simulink model "btp_VERSION2_final"  (R2020a)
settings: Solver=VariableStepAuto  StartTime=0.0  StopTime=14000  RelTol=1e-3
PreLoadFcn:
  | building_length = 15; % m
  | building_width = 10; % m
  | building_height = 2.5; % m
  | 
  | wall_thickness = 0.2; % m
  | wall_density = 2000; % kg/m^3
  | wall_specific_heat = 840; % J/(kg*K)
  | wall_conductivity = 0.04; % W/(m*K)
  | wall_heat_transfer_coeff_internal = 25; % W/(m^2*K)
  | wall_heat_transfer_coeff_external = 35; % W/(m^2*K)
  | 
  | roof_thickness = 0.2; % m
  | roof_density = 2000; % kg/m^3
  | roof_specific_heat = 840; % J/(kg*K)
  | roof_conductivity = 0.035; % W/(m*K)
  | roof_heat_transfer_coeff_internal = 10; % W/(m^2*K)
  | roof_heat_transfer_coeff_external = 30; % W/(m^2*K)
  | 
  | floor_thickness = 0.1; % m
  | floor_conductivity = 0.15; % W/(m*K)
  | floor_heat_transfer_coeff_internal = 15; % W/(m^2*K)
  | 
  | door_area = 2*0.6; % m^2
  | 
  | duct_area = 0.1^2; % m^2
  | 
  | fan_setting_table = 0 : 4; % 1
  | fan_flow_rate_table = [0 0.08 0.12 0.16 0.2]; % kg/s
  | 
  | initial_temperature = 35; % degC
  | ground_temperature = 25; % degC
  | 
  | flow_reversal_Mach = 1e-5; % 1
InitFcn:
  | zone_volume = building_length * building_width * building_height / 4; % m^3
  | zone_flow_area = 0.7 * building_height * (building_length + building_width) / 4; % m^2
model workspace (MAT data in the model file):
  building_height = 3
  building_length = 4.4
  building_width = 4
  door_area = Simulink.Parameter
  door_area.Value = 2
  door_area.DataType = 'double'
  door_area.Dimensions = [1 1]
  duct_area = 0.02
  fan_flow_rate_table = [0 0.08 0.12 0.16 0.2]
  fan_setting_table = [0 1 2 3 4]
  floor_conductivity = 0.15
  floor_heat_transfer_coeff_internal = 15
  floor_thickness = 0.1
  flow_reversal_Mach = 1e-05
  ground_temperature = 27
  initial_temperature = 35
  roof_conductivity = 0.04
  roof_density = 2000
  roof_heat_transfer_coeff_external = 30
  roof_heat_transfer_coeff_internal = 10
  roof_specific_heat = 840
  roof_thickness = 0.2
  simlog_ssc_building_ventilation : simscape.logging.Node (value not decoded)
  tout = [0 3.15544362088e-30 8.45959628835e-09 2.5378788865e-08 3.73619145974e-08 4.93450403297e-08 6.73197289282e-08 8.52944175267e-08 1.12256450424e-07 1.39218483322e-07 1.6618051622e-07 1.93142549118e-07 ... (463 elements, 463x1)]
  wall_conductivity = 0.04
  wall_density = 2000
  wall_heat_transfer_coeff_external = 35
  wall_heat_transfer_coeff_internal = 25
  wall_specific_heat = 840
  wall_thickness = 0.2
  zone_flow_area = 9
  zone_volume = 50
undefined symbols (not defined in the file): dbresponses22S1, sigbuilder_block
libraries: fl_lib x53, nesl_utility x27, HVAC_lib x2, simulink x2, fuzblock x1
(part 1 of 2)
CloseFcn:
  | try,close(h1_ssc_building_ventilation),end
  | clear h1_ssc_building_ventilation
  | try,close(h2_ssc_building_ventilation),end
  | clear h2_ssc_building_ventilation
  | try,close(h3_ssc_building_ventilation),end
  | clear h3_ssc_building_ventilation
  | try,close(h4_ssc_building_ventilation),end
  | clear h4_ssc_building_ventilation
  | 
  | clear simlog_ssc_building_ventilation tout
  | 
  | clear building_length building_width building_height zone_volume zone_flow_area
  | clear wall_thickness wall_density wall_specific_heat wall_conductivity wall_heat_transfer_coeff_internal wall_heat_transfer_coeff_external
  | clear roof_thickness roof_density roof_specific_heat roof_conductivity roof_heat_transfer_coeff_internal roof_heat_transfer_coeff_external
  | clear floor_thickness floor_conductivity floor_heat_transfer_coeff_internal
  | clear door_area duct_area fan_setting_table fan_flow_rate_table initial_temperature ground_temperature flow_reversal_Mach
Description:
  | Building Ventilation
settings Model: OrderedModelArguments=off  Creator=MathWorks  LastModifiedBy=PRANAV REDDY
settings DataIOCC: ReturnWorkspaceOutputs=off
settings DebuggingCC: PregeneratedLibrarySubsystemCodeDiagnostic=none  ArithmeticOperatorsInVariantConditions=warning
settings SFSimCC: SimUseLocalCustomCode=off  CustomCodeUndefinedFunction=UseInterfaceOnly
settings RTWCC: RTWUseLocalCustomCode=off
settings CodeAppCC: StateflowObjectComments=on
settings SimscapeCC: SimscapeLogType=all  SimscapeLogSimulationStatistics=on  SimscapeLogName=simlog_ssc_building_ventilation  SimscapeLogDataHistory=10000

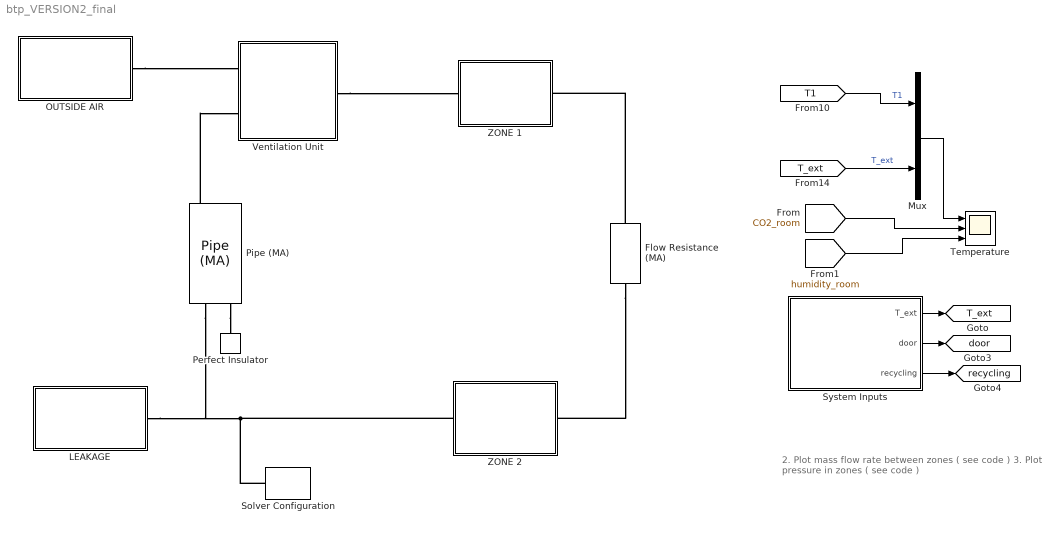
== system btp_VERSION2_final ==
  note: 2. Plot mass flow rate between zones ( see code )
      | 3. Plot pressure in zones ( see code )
  Flow Resistance (MA) : fl_lib/Moist Air/Elements/Flow Resistance (MA)  delta_p_nominal=10 Pa  mdot_nominal=0.45 kg/s  rho_nominal=1.2 kg/m^3  area=zone_flow_area m^2  laminar_fraction=1e-3
      settings: SourceProductBaseCode=SS
  LEAKAGE : Subsystem
  Mux : Mux  Inputs=2
  OUTSIDE AIR : Subsystem
  Perfect Insulator : fl_lib/Thermal/Thermal Elements/Perfect Insulator  T_specify=off  T_priority=None  T=0 K  T_nominal_specify=off  T_nominal_unit=K  T_nominal_value=1
  Pipe (MA) : fl_lib/Moist Air/Elements/Pipe (MA)  length=building_length + building_width m  area=duct_area m^2  Dh=sqrt(duct_area) m  length_add=0 m  roughness=15e-6 m  Re_lam=2000  Re_tur=4000  shape_factor=56.92  Nu_lam=2.98  RH_ws=1  time_constant=1e-3 s  moisture_trace_gas_source=foundation.enum.moisture_trace_gas_source.none  moisture_source_spec=foundation.enum.moisture_source_spec.vapor  moisture_mass_flow=0 kg/s  moisture_temperature_spec=foundation.enum.temperature_spec.atmospheric  moisture_temperature=293.15 K  trace_gas_mass_flow=0 kg/s  trace_gas_temperature_spec=foundation.enum.temperature_spec.atmospheric  trace_gas_temperature=293.15 K  p_I_specify=on  p_I_priority=High  p_I=0.101325 MPa  p_I_nominal_specify=off  p_I_nominal_unit=MPa  p_I_nominal_value=1  T_I_specify=off  T_I_priority=None  T_I=initial_temperature K  T_I_nominal_specify=off  T_I_nominal_unit=K  T_I_nominal_value=1  RH_I_specify=on  RH_I_priority=None  RH_I=0.57  RH_I_nominal_specify=off  RH_I_nominal_unit=1  RH_I_nominal_value=1  x_w_I_specify=off  x_w_I_priority=None  x_w_I=0  x_w_I_nominal_specify=off  x_w_I_nominal_unit=1  x_w_I_nominal_value=1  y_w_I_specify=off  y_w_I_priority=None  y_w_I=0  y_w_I_nominal_specify=off  y_w_I_nominal_unit=1  y_w_I_nominal_value=1  HR_I_specify=off  HR_I_priority=None  HR_I=0  HR_I_nominal_specify=off  HR_I_nominal_unit=1  HR_I_nominal_value=1  x_g_I_specify=off  x_g_I_priority=High  x_g_I=0  x_g_I_nominal_specify=off  x_g_I_nominal_unit=1  x_g_I_nominal_value=1  y_g_I_specify=on  y_g_I_priority=None  y_g_I=0.00045  y_g_I_nominal_specify=off  y_g_I_nominal_unit=1  y_g_I_nominal_value=1
      settings: SourceProductBaseCode=SS
  Solver Configuration : nesl_utility/Solver Configuration  PhysicalDomain=network_engine_domain  SubClassName=solver  LeftPortType=input  RightPortType=generic  Tones=[]  Harmonics=[]  SimulateNoise=off  Profile=off  UseLocalSampling=off  EnableSwitchedLinearOptims=on  FrequencyDomain=off  UseCCode=off  RelTol=0.001  AbsTol=1e-06  MinStep=1e-09  ToWorkspace=off  RevertToSquareIcSolve=off  NumHomotopyIterations=100  PhasorMode=off  PhasorModeNumHarmonics=1  DoDC=off  ResidualTolerance=1e-9  UseLocalSolver=off  LocalSolverChoice=NE_BACKWARD_EULER_ADVANCER  LocalSolverSampleTime=0.05  DoFixedCost=off  MaxNonlinIter=3  MaxModeIter=2  LinearAlgebra=auto  EquationFormulation=NE_TIME_EF  DelaysMemoryBudget=1024  AutomaticFiltering=on  FilteringTimeConstant=0.001  PartitionStorageMethod=AS_NEEDED  PartitionMemoryBudget=1024  PartitionMethod=FAST
  System Inputs : Subsystem  Tag=STV Subsys  LoadFcn=sigbuilder_block('load');  StartFcn=sigbuilder_block('start');  StopFcn=sigbuilder_block('stop');  ClipboardFcn=sigbuilder_block('clipboard');  mask(Sigbuilder block){tuvar=[0:10]}
      mask help: Simulink:masks:SigbuilderBlock_MD
      mask init:
      | if ~strcmp(get_param(bdroot(gcbh),'SimulationStatus'),'stopped') tuvar = sigbuilder_block('maskInit'); end
      settings: CopyFcn=sigbuilder_block('copy');  DeleteFcn=sigbuilder_block('delete');  ModelCloseFcn=sigbuilder_block('modelClose');  PreSaveFcn=sigbuilder_block('preSave');  PauseFcn=sigbuilder_block('pause');  ContinueFcn=sigbuilder_block('continue');  NameChangeFcn=sigbuilder_block('namechange');  OpenFcn=sigbuilder_block('open',[398.25 64.5 506.25 359.25 ]);  CloseFcn=sigbuilder_block('close');
      mask Display: plot(0, 0, 100, 100,[2, 2, 32, 32, 2], [68, 8, 8, 68, 68],[32, 2], [38, 38], [32, 19, 2],[53, 60, 44], [32, 17, 17, 2],[16, 16, 31, 31]);txt = getActiveGroup(gcbh);text(2, 100, txt,'verticalAlignment', 'top');
  Temperature : Scope  NumInputPorts=3
  Ventilation Unit : Subsystem  Tag=PublishSubsystem
  ZONE 1 : Subsystem
  ZONE 2 : Subsystem
  tag scope: T_ext=global, door=global, recycling=global
  wires:
  System Inputs/1(T_ext) -> [T_ext]
  System Inputs/2(door) -> [door]
  System Inputs/3(recycling) -> [recycling]
  [T1] -> Mux/1  "T1"
  [T_ext] -> Mux/2  "T_ext"
  Mux/1 -> Temperature/1
  [CO2_room] -> Temperature/2
  [humidity_room] -> Temperature/3
  connections:
  Pipe (MA)/RConn1 -- Ventilation Unit/LConn2
  Pipe (MA)/LConn2 -- Perfect Insulator/LConn1
  Solver Configuration/RConn1 -- LEAKAGE/RConn1 -- Pipe (MA)/LConn1 -- ZONE 2/LConn1
  OUTSIDE AIR/RConn1 -- Ventilation Unit/LConn1
  Flow Resistance (MA)/LConn1 -- ZONE 1/RConn1
  Flow Resistance (MA)/RConn1 -- ZONE 2/RConn1
  Ventilation Unit/RConn1 -- ZONE 1/LConn1

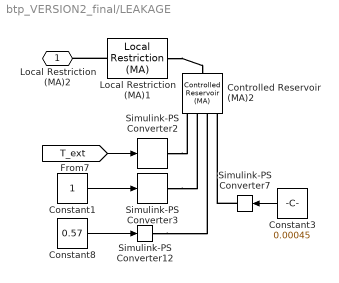
== system btp_VERSION2_final/LEAKAGE ==
  Constant1 : Constant
  Constant3 : Constant  Value=0.00045
  Constant8 : Constant  Value=0.57
  Controlled Reservoir (MA)2 : fl_lib/Moist Air/Elements/Controlled Reservoir (MA)  moisture_spec=foundation.enum.moisture_spec.relative_humidity  trace_gas_spec=foundation.enum.trace_gas_spec.mole_fraction  RH_ws=1  area_A=duct_area m^2  input_error_spec=foundation.enum.input_range_error.warn
      settings: SourceProductBaseCode=SS  InternalSimscapePortConfiguration="{\"Bottom\":[],\"Left\":[{\"id\":\"A\",\"label\":\"A\",\"type\":\"foundation.moist_air.moist_air\"}],\"Right\":[{\"id\":\"T\",\"label\":\"T\",\"type\":\"input\"},{\"id\":\"P\",\"label\":\"P\",\"type\":\"input\"},{\"id\":\"W\",\"label\":\"W\",\"type\":\"input\"},{\"id\":\"G\",\"label\":\"G\",\"type\":\"input\"}],\"Top\":[]}"
  Local Restriction (MA)1 : fl_lib/Moist Air/Elements/Local Restriction (MA)  restriction_type=foundation.enum.restriction_type.fixed  restriction_area=0.4 * duct_area m^2  min_area=1e-10 m^2  max_area=0.5*duct_area m^2  area=0.8*duct_area m^2  Cd=0.8  B_lam=0.999
      settings: SourceProductBaseCode=SS  InternalSimscapePortConfiguration="{\"Bottom\":[],\"Left\":[{\"id\":\"A\",\"label\":\"A\",\"type\":\"foundation.moist_air.moist_air\"}],\"Right\":[{\"id\":\"B\",\"label\":\"B\",\"type\":\"foundation.moist_air.moist_air\"}],\"Top\":[]}"
  Simulink-PS Converter12 : nesl_utility/Simulink-PS Converter  PhysicalDomain=network_engine_domain  SubClassName=ps_input  LeftPortType=input  RightPortType=output  PseudoPeriodic=off  Frequencies=[]  NoiseDistribution=none  NoiseParameters=[]  Unit=1  AffineConversion=off  FilteringAndDerivatives=provide  SimscapeFilterOrder=1  InputFilterTimeConstant=0.001  UdotUserProvided=0
  Simulink-PS Converter2 : nesl_utility/Simulink-PS Converter  PhysicalDomain=network_engine_domain  SubClassName=ps_input  LeftPortType=input  RightPortType=output  PseudoPeriodic=off  Frequencies=[]  NoiseDistribution=none  NoiseParameters=[]  Unit=degC  AffineConversion=on  FilteringAndDerivatives=provide  SimscapeFilterOrder=1  InputFilterTimeConstant=0.001  UdotUserProvided=0
  Simulink-PS Converter3 : nesl_utility/Simulink-PS Converter  PhysicalDomain=network_engine_domain  SubClassName=ps_input  LeftPortType=input  RightPortType=output  PseudoPeriodic=off  Frequencies=[]  NoiseDistribution=none  NoiseParameters=[]  Unit=atm  AffineConversion=off  FilteringAndDerivatives=provide  SimscapeFilterOrder=1  InputFilterTimeConstant=0.001  UdotUserProvided=0
  Simulink-PS Converter7 : nesl_utility/Simulink-PS Converter  PhysicalDomain=network_engine_domain  SubClassName=ps_input  LeftPortType=input  RightPortType=output  PseudoPeriodic=off  Frequencies=[]  NoiseDistribution=none  NoiseParameters=[]  Unit=1  AffineConversion=off  FilteringAndDerivatives=provide  SimscapeFilterOrder=1  InputFilterTimeConstant=0.001  UdotUserProvided=0
  Local Restriction (MA)2 : PMIOPort  Side=Right
  wires:
  Constant3/1 -> Simulink-PS Converter7/1
  Constant8/1 -> Simulink-PS Converter12/1
  [T_ext] -> Simulink-PS Converter2/1
  Constant1/1 -> Simulink-PS Converter3/1
  connections:
  Simulink-PS Converter2/RConn1 -- Controlled Reservoir (MA)2/RConn1
  Simulink-PS Converter12/RConn1 -- Controlled Reservoir (MA)2/RConn3
  Local Restriction (MA)1/RConn1 -- Controlled Reservoir (MA)2/LConn1
  Simulink-PS Converter7/RConn1 -- Controlled Reservoir (MA)2/RConn4
  Simulink-PS Converter3/RConn1 -- Controlled Reservoir (MA)2/RConn2
  Local Restriction (MA)1/LConn1 -- Local Restriction (MA)2/RConn1

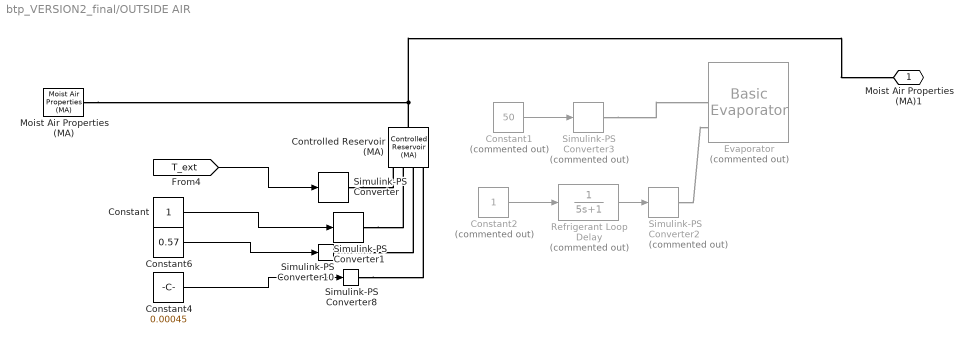
== system btp_VERSION2_final/OUTSIDE AIR ==
  Constant : Constant
  Constant1 : Constant  Commented=on  Value=50
  Constant2 : Constant  Commented=on
  Constant4 : Constant  Value=0.00045
  Constant6 : Constant  Value=0.57
  Controlled Reservoir (MA) : fl_lib/Moist Air/Elements/Controlled Reservoir (MA)  moisture_spec=foundation.enum.moisture_spec.relative_humidity  trace_gas_spec=foundation.enum.trace_gas_spec.mole_fraction  RH_ws=1  area_A=duct_area m^2  input_error_spec=foundation.enum.input_range_error.warn
      settings: SourceProductBaseCode=SS  InternalSimscapePortConfiguration="{\"Bottom\":[],\"Left\":[{\"id\":\"A\",\"label\":\"A\",\"type\":\"foundation.moist_air.moist_air\"}],\"Right\":[{\"id\":\"T\",\"label\":\"T\",\"type\":\"input\"},{\"id\":\"P\",\"label\":\"P\",\"type\":\"input\"},{\"id\":\"W\",\"label\":\"W\",\"type\":\"input\"},{\"id\":\"G\",\"label\":\"G\",\"type\":\"input\"}],\"Top\":[]}"
  Evaporator : HVAC_lib/Basic Evaporator  Commented=on  Q_des=3 kW  T1_des=30 degC  mdot1_des=0.1 kg/s  cp1_des=1.006 kJ/kg/K  Dp1_des=0.2 kPa  T2_des=85 degC  mdot2_des=1 kg/s  volume=2e-1 m^3  port_area=duct_area m^2  RH_ws=1  time_constant=1e-3 s  p_I_specify=off  p_I_priority=High  p_I=p_env MPa  p_I_nominal_specify=off  p_I_nominal_unit=MPa  p_I_nominal_value=1  T_I_specify=on  T_I_priority=High  T_I=initial_temperature degC  T_I_nominal_specify=off  T_I_nominal_unit=K  T_I_nominal_value=1  RH_I_specify=on  RH_I_priority=High  RH_I=0.57  RH_I_nominal_specify=off  RH_I_nominal_unit=1  RH_I_nominal_value=1  x_w_I_specify=off  x_w_I_priority=None  x_w_I=0  x_w_I_nominal_specify=off  x_w_I_nominal_unit=1  x_w_I_nominal_value=1  y_w_I_specify=off  y_w_I_priority=None  y_w_I=0  y_w_I_nominal_specify=off  y_w_I_nominal_unit=1  y_w_I_nominal_value=1  HR_I_specify=off  HR_I_priority=None  HR_I=0  HR_I_nominal_specify=off  HR_I_nominal_unit=1  HR_I_nominal_value=1  x_g_I_specify=off  x_g_I_priority=None  x_g_I=0  x_g_I_nominal_specify=off  x_g_I_nominal_unit=1  x_g_I_nominal_value=1  y_g_I_specify=on  y_g_I_priority=High  y_g_I=0.00045  y_g_I_nominal_specify=off  y_g_I_nominal_unit=1  y_g_I_nominal_value=1
      settings: SourceProductBaseCode=SS  InternalSimscapePortConfiguration="{\"Bottom\":[],\"Left\":[{\"id\":\"A\",\"label\":\"A\",\"type\":\"foundation.moist_air.moist_air\"},{\"id\":\"T2\",\"label\":\"T2\",\"type\":\"input\"},{\"id\":\"M2\",\"label\":\"M2\",\"type\":\"input\"}],\"Right\":[{\"id\":\"B\",\"label\":\"B\",\"type\":\"foundation.moist_air.moist_air\"},{\"id\":\"W\",\"label\":\"W\",\"type\":\"output\"},{\"id\":\"F\",\"label\":\"F\",\"type\":\"output\"}],\"Top\":[]}"
  Moist Air Properties (MA) : fl_lib/Moist Air/Utilities/Moist Air Properties (MA)  trace_gas_model=2  R_a=287.047 J/kg/K  R_w=461.523 J/kg/K  R_g=188.923 J/kg/K  T_TLU=[-56.55, -50 : 10 : -10, -5 : 1 : 5, 10 : 10 : 350]' degC  p_ws_TLU=[1.71168953425982e-06; 3.93770601979424e-06; 1.28411717710344e-05; 3.80051394873809e-05; .00010323902900209; .000259873810798063; .000401741022116384; .000437454836117844; .000476040820618202; .000517704666185737; .000562664883741207; .000611212677444345; .000657088049117899; .000705987905898279; .000758082381149132; .000813549384183233; .000872574861129522; .00122818386934022; .0023392147667769; .00424668834054807; .00738442748706953; .0123512704340234; .0199458019246787; .0312006356960619; .0474147199263783; .0701823607447713; .10141797792131; .143375967241115; .198665399739302; .270259606559999; .361500961984849; .476101381081492; .618139196722055; .792053183687694; 1.0026345688121; 1.25501792086105; 1.55467186826983; 1.90739066433297; 2.31928772772542; 2.79679245576864; 3.34665187151016; 3.97593907083533; 4.69207105435535; 5.5028394740883; 6.41645928168037; 7.4416425436169; 8.58770832955728; 9.86474556030261; 11.2838558865497; 12.8575218898034; 14.6001810568052; 16.5291642526045] MPa  h_w_vap_TLU=[2836.88241275372; 2837.81392500514; 2838.63937175807; 2838.7309929628; 2838.06905313927; 2836.62597341095; 2835.60023952573; 2835.37006381376; 2835.13143158077; 2834.88429145066; 2834.62859062897; 2500.93420564316; 2498.55329907119; 2496.17495082036; 2493.79885912205; 2491.42474723191; 2489.05236104642; 2477.20875029194; 2453.54955988604; 2429.83856603313; 2406.00136954922; 2381.97406342174; 2357.69101156389; 2333.08088387814; 2308.06565480412; 2282.56034405021; 2256.47287422313; 2229.70428017508; 2202.14968030993; 2173.69998896199; 2144.24368406447; 2113.66758247452; 2081.85585110571; 2048.68725710494; 2014.03141249899; 1977.7449923284; 1939.66849592886; 1899.62342931686; 1857.40930169838; 1812.79975416601; 1765.53721731251; 1715.32525772152; 1661.81700477787; 1604.59703745016; 1543.1534616334; 1476.83692476464; 1404.80240352424; 1325.92091736114; 1238.61667822208; 1140.5102987018; 1027.62017777647; 892.733785613825] kJ/kg  h_a_TLU=[342.416126230579; 349.005511058471; 359.063577249119; 369.119948684177; 379.175469465129; 389.230944678417; 394.258910928084; 395.264534937366; 396.27017101329; 397.275819932805; 398.281482472874; 399.287159410541; 400.292851523015; 401.298559587728; 402.304284382408; 403.310026685143; 404.315787274435; 409.34489180313; 419.404921755863; 429.468036401264; 439.535033154839; 449.606720928652; 459.683919949603; 469.767460521911; 479.858181001348; 489.956925196484; 500.064539372946; 510.181869006204; 520.309755403634; 530.449032296018; 540.60052248087; 550.765034584465; 560.943359995745; 571.136270013102; 581.344513234296; 591.568813210327; 601.809866375885; 612.068340261954; 622.344871990218; 632.640067043998; 642.95449830646; 653.288705353699; 663.643193987949; 674.018435994423; 684.414869104228; 694.832897145098; 705.272890361557; 715.735185886199; 726.220088344236; 736.727870574087; 747.258774447567; 757.813011774199] kJ/kg  h_w_TLU=[2396.55944251649; 2408.68643343608; 2427.1988031141; 2445.702165897; 2464.18429108356; 2482.62529466839; 2491.82135326629; 2493.6580151792; 2495.49372578218; 2497.32843835745; 2499.16210446923; 2500.99462758899; 2502.83092214066; 2504.6665223621; 2506.50140563013; 2508.335548891; 2510.16892865793; 2519.32352241995; 2537.56068088674; 2555.67742615292; 2573.6403223998; 2591.4109179101; 2608.9455037701; 2626.19492016262; 2643.10444358428; 2659.61377634497; 2675.58278696023; 2696.1846256545; 2716.49989553741; 2736.6235210957; 2756.61216047011; 2776.50561773853; 2796.33378922508; 2816.11979583049; 2835.88181423877; 2855.63430574511; 2875.38889327595; 2895.15500577172; 2914.94035964689; 2934.75132290228; 2954.59319330244; 2974.47041285505; 2994.38673458964; 3014.34535328009; 3034.34900867103; 3054.40006755764; 3074.50058946898; 3094.65237953784; 3114.85703128106; 3135.11596137801; 3155.43043805905; 3175.80160435813] kJ/kg  h_g_TLU=[439.555216260064; 444.670268200251; 452.538618847003; 460.487124258496; 468.522588768941; 476.649415958793; 480.74798538725; 481.57054318762; 482.394052398751; 483.218514288831; 484.043930029015; 484.870300696555; 485.697627277859; 486.525910671489; 487.355151691079; 488.185351068185; 489.016509455051; 493.186704139431; 501.599194953048; 510.107689961685; 518.711611080182; 527.410026793075; 536.201764778798; 545.085474203452; 554.059675505208; 563.122805485367; 572.27325096919; 581.509373027928; 590.829525105886; 600.232066705818; 609.715373581392; 619.277845178105; 628.917909922924; 638.634028838794; 648.424697859328; 658.288449140109; 668.223851601449; 678.229510889093; 688.304068901113; 698.44620299875; 708.654624994591; 718.928079991818; 729.265345132425; 739.665228299475; 750.126566808087; 760.648226111439; 771.229098541268; 781.868102096908; 792.564179292476; 803.316296068366; 814.123440770426; 824.984623198037] kJ/kg  mu_a_TLU=[14.2568883320012; 14.6140127728333; 15.1517277055779; 15.6806860159119; 16.2012351072083; 16.7137043125028; 16.9670071730589; 17.017438062815; 17.0677930842452; 17.1180725309876; 17.1682766951315; 17.2184058672268; 17.2684603362935; 17.3184403898301; 17.3683463138234; 17.4181783927569; 17.4679369096204; 17.7156358640698; 18.2056751785154; 18.68879035749; 19.1652344664982; 19.6352478927873; 20.099059103658; 20.5568853601578; 21.0089333871663; 21.4554000014051; 21.8964726992323; 22.3323302062775; 22.7631429910631; 23.1890737447833; 23.6102778293792; 24.0269036959922; 24.4390932757886; 24.8469823450548; 25.2507008663546; 25.6503733074314; 26.0461189394339; 26.4380521159325; 26.8262825340948; 27.2109154792923; 27.5920520543128; 27.969789394274; 28.3442208682439; 28.7154362685068; 29.0835219883356; 29.4485611890712; 29.8106339572472; 30.1698174524429; 30.5261860464955; 30.8798114546565; 31.2307628592324; 31.5791070262086] s*uPa  mu_w_TLU=[6.81365662228272; 7.04953750742707; 7.40970098298307; 7.76991278093907; 8.13017290129507; 8.49048134405107; 8.67065368632907; 8.70668960445667; 8.74272600580827; 8.77876289038387; 8.81480025818347; 8.85083810920707; 8.88687644345467; 8.92291526092627; 8.95895456162187; 8.99499434554147; 9.03103461268507; 9.21124319676307; 9.57169660671907; 9.93219833907507; 10.2927483938311; 10.6533467709871; 11.0139934705431; 11.3746884924991; 11.7354318368551; 12.0962235036111; 12.4570634927671; 12.8179518043231; 13.1788884382791; 13.5398733946351; 13.9009066733911; 14.2619882745471; 14.6231181981031; 14.9842964440591; 15.3455230124151; 15.7067979031711; 16.0681211163271; 16.4294926518831; 16.7909125098391; 17.1523806901951; 17.5138971929511; 17.8754620181071; 18.2370751656631; 18.5987366356191; 18.9604464279751; 19.3222045427311; 19.6840109798871; 20.0458657394431; 20.4077688213991; 20.7697202257551; 21.1317199525111; 21.4937680016671] s*uPa  mu_g_TLU=[10.8921054191698; 11.2215357085649; 11.7233300740382; 12.2234238147811; 12.7215124453467; 13.2173328890673; 13.4643203184773; 13.5136406274989; 13.562934752385; 13.6122025024997; 13.6614436900741; 13.7106581301692; 13.7598456406398; 13.8090060420983; 13.8581391578796; 13.9072448140062; 13.9563228391538; 14.2012926853717; 14.6890687376044; 15.1738428124161; 15.6554929043332; 16.1339159800463; 16.6090257998657; 17.0807510097148; 17.5490334645512; 18.0138267508952; 18.4750948814453; 18.9328111390399; 19.3869570507278; 19.8375214755778; 20.2844997922255; 20.7278931741254; 21.1677079421287; 21.6039549853963; 22.036649242835; 22.4658092382469; 22.8914566632375; 23.3136160026627; 23.7323141980278; 24.1475803447965; 24.5594454200432; 24.9679420372927; 25.3731042257492; 25.774967231431; 26.1735673380029; 26.5689417053362; 26.9611282240413; 27.350165384404; 27.73609215832; 28.118947892972; 28.4987722151178; 28.8756049449796] s*uPa  k_a_TLU=[19.8808489374933; 20.4162454629695; 21.2248743590758; 22.0232452890903; 22.8117314495857; 23.5906913619588; 23.9767075412237; 24.053639990175; 24.1304826682191; 24.2072359051629; 24.2839000294007; 24.3604753679152; 24.4369622462801; 24.5133609886625; 24.5896719178249; 24.6658953551279; 24.7420316205333; 25.1214164701832; 25.8738283029331; 26.6180150229276; 27.3542674377332; 28.0828634735341; 28.8040686837224; 29.5181367785657; 30.2253101618423; 30.9258204644224; 31.6198890677835; 32.3077276126633; 32.9895384896798; 33.6655153099498; 34.33584335461; 35.0007000027879; 35.6602551380254; 36.3146715334901; 36.9641052165342; 37.6087058133173; 38.248616874307; 38.8839761815308; 39.5149160384798; 40.1415635435708; 40.7640408480637; 41.3824653993118; 41.9969501701893; 42.6076038755117; 43.2145311762238; 43.8178328720941; 44.4176060836121; 45.013944423749; 45.6069381602018; 46.1966743687041; 46.783237077953; 47.3667074066625] mW/m/K  k_w_TLU=[11.46288215976; 11.941997488935; 12.676358586935; 13.414208884935; 14.155548382935; 14.900377080935; 15.274099879935; 15.348949115735; 15.423833243535; 15.498752263335; 15.573706175135; 15.648694978935; 15.723718674735; 15.798777262535; 15.873870742335; 15.948999114135; 16.024162377935; 16.400502076935; 17.155798374935; 17.914583872935; 18.676858570935; 19.442622468935; 20.211875566935; 20.984617864935; 21.760849362935; 22.540570060935; 23.323779958935; 24.110479056935; 24.900667354935; 25.694344852935; 26.491511550935; 27.292167448935; 28.096312546935; 28.903946844935; 29.715070342935; 30.529683040935; 31.347784938935; 32.169376036935; 32.994456334935; 33.823025832935; 34.655084530935; 35.490632428935; 36.329669526935; 37.172195824935; 38.018211322935; 38.867716020935; 39.720709918935; 40.577193016935; 41.437165314935; 42.300626812935; 43.167577510935; 44.038017408935] mW/m/K  k_g_TLU=[10.489430678843; 10.9507672150864; 11.666197960308; 12.392559739764; 13.1299519771612; 13.8778409888416; 14.2554325416312; 14.3312274189707; 14.4071122346908; 14.4830860227061; 14.5591478179508; 14.6352966574703; 14.7115315815553; 14.787851634907; 14.8642558678259; 14.9407433374142; 15.0173131087819; 15.401364480906; 16.1751373988038; 16.9558134611595; 17.7432208682398; 18.5366976599676; 19.3360988502003; 20.1412225692689; 20.9517507672929; 21.7672310558863; 22.5871115634685; 23.4107980865695; 24.2377021890869; 25.0672663781241; 25.8989689893876; 26.732318357514; 27.5668446164644; 28.4020933015927; 29.2376215872816; 30.0729965057542; 30.9077942826816; 31.7416001931033; 32.5740086297993; 33.4046232539953; 34.2330571812868; 35.0589331874899; 35.8818839295189; 36.701552179391; 37.5175910702657; 38.3296643536716; 39.1374466671854; 39.9406238119064; 40.7388930391313; 41.5319633456945; 42.3195557774861; 43.1014037407076] mW/m/K  D_w=25 mm^2/s  D_g=16 mm^2/s  p_min=1 kPa  p_max=inf MPa  T_min=-56.55 degC  T_max=350 degC  p_atm=0.101325 MPa  T_atm=20 degC
      settings: SourceProductBaseCode=SS
  Refrigerant Loop Delay : TransferFcn  Commented=on  Denominator=[5 1]
  Simulink-PS Converter : nesl_utility/Simulink-PS Converter  PhysicalDomain=network_engine_domain  SubClassName=ps_input  LeftPortType=input  RightPortType=output  PseudoPeriodic=off  Frequencies=[]  NoiseDistribution=none  NoiseParameters=[]  Unit=degC  AffineConversion=on  FilteringAndDerivatives=provide  SimscapeFilterOrder=1  InputFilterTimeConstant=0.001  UdotUserProvided=0
  Simulink-PS Converter1 : nesl_utility/Simulink-PS Converter  PhysicalDomain=network_engine_domain  SubClassName=ps_input  LeftPortType=input  RightPortType=output  PseudoPeriodic=off  Frequencies=[]  NoiseDistribution=none  NoiseParameters=[]  Unit=atm  AffineConversion=off  FilteringAndDerivatives=provide  SimscapeFilterOrder=1  InputFilterTimeConstant=0.001  UdotUserProvided=0
  Simulink-PS Converter10 : nesl_utility/Simulink-PS Converter  PhysicalDomain=network_engine_domain  SubClassName=ps_input  LeftPortType=input  RightPortType=output  PseudoPeriodic=off  Frequencies=[]  NoiseDistribution=none  NoiseParameters=[]  Unit=1  AffineConversion=off  FilteringAndDerivatives=provide  SimscapeFilterOrder=1  InputFilterTimeConstant=0.001  UdotUserProvided=0
  Simulink-PS Converter2 : nesl_utility/Simulink-PS Converter  Commented=on  PhysicalDomain=network_engine_domain  SubClassName=ps_input  LeftPortType=input  RightPortType=output  PseudoPeriodic=off  Frequencies=[]  NoiseDistribution=none  NoiseParameters=[]  Unit=kg/s  AffineConversion=on  FilteringAndDerivatives=provide  SimscapeFilterOrder=1  InputFilterTimeConstant=0.001  UdotUserProvided=0
  Simulink-PS Converter3 : nesl_utility/Simulink-PS Converter  Commented=on  PhysicalDomain=network_engine_domain  SubClassName=ps_input  LeftPortType=input  RightPortType=output  PseudoPeriodic=off  Frequencies=[]  NoiseDistribution=none  NoiseParameters=[]  Unit=degC  AffineConversion=on  FilteringAndDerivatives=provide  SimscapeFilterOrder=1  InputFilterTimeConstant=0.001  UdotUserProvided=0
  Simulink-PS Converter8 : nesl_utility/Simulink-PS Converter  PhysicalDomain=network_engine_domain  SubClassName=ps_input  LeftPortType=input  RightPortType=output  PseudoPeriodic=off  Frequencies=[]  NoiseDistribution=none  NoiseParameters=[]  Unit=1  AffineConversion=off  FilteringAndDerivatives=provide  SimscapeFilterOrder=1  InputFilterTimeConstant=0.001  UdotUserProvided=0
  Moist Air Properties (MA)1 : PMIOPort  Side=Right
  wires:
  Constant4/1 -> Simulink-PS Converter8/1
  Constant6/1 -> Simulink-PS Converter10/1
  [T_ext] -> Simulink-PS Converter/1
  Constant/1 -> Simulink-PS Converter1/1
  Refrigerant Loop Delay/1 -> Simulink-PS Converter2/1
  Constant2/1 -> Refrigerant Loop Delay/1
  Constant1/1 -> Simulink-PS Converter3/1
  connections:
  Simulink-PS Converter10/RConn1 -- Controlled Reservoir (MA)/RConn3
  Simulink-PS Converter8/RConn1 -- Controlled Reservoir (MA)/RConn4
  Simulink-PS Converter/RConn1 -- Controlled Reservoir (MA)/RConn1
  Simulink-PS Converter1/RConn1 -- Controlled Reservoir (MA)/RConn2
  Simulink-PS Converter3/RConn1 -- Evaporator/LConn2
  Simulink-PS Converter2/RConn1 -- Evaporator/LConn3
  Controlled Reservoir (MA)/LConn1 -- Moist Air Properties (MA)1/RConn1 -- Moist Air Properties (MA)/RConn1

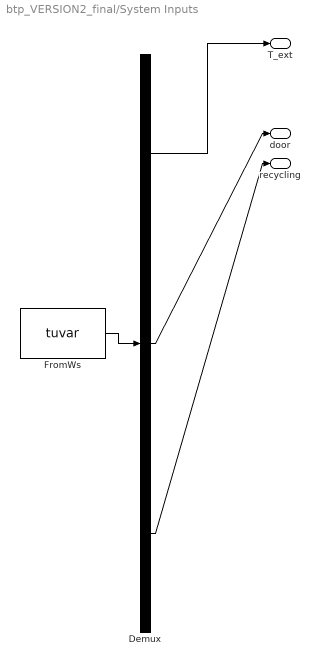
== system btp_VERSION2_final/System Inputs ==
  Demux : Demux  Tag=STV Demux  Outputs=3
      settings: DisplayOption=none
  FromWs : FromWorkspace  Tag=STV FromWs  VariableName=tuvar
      SigBuilderData=|
      | common.afterFinalStr = 'Extrapolate'
      | common.sampleTime = 0
      | dataSet(1).timeRange = [0 14000]
      | dataSet(1).name = 'Fan Control'
      | dataSet(2).timeRange = [0 100000]
      | dataSet(2).name = 'Fan Temperature'
      | dataSet(3).timeRange = [0 100000]
      | dataSet(3).name = 'Disturbances'
      | sbobj.Groups(1).Name = 'Fan Control'
      | sbobj.Groups(1).Signals(1).Name = 'T_ext'
      | sbobj.Groups(1).Signals(1).XData = [0 5510 5700 7800 8900 14000]
      | sbobj.Groups(1).Signals(1).YData = [35 35 35 35 35 32.5]
      | sbobj.Groups(1).Signals(2).Name = 'door'
      | sbobj.Groups(1).Signals(2).XData = [0 3950 3950 4350 4350 14000]
      | sbobj.Groups(1).Signals(2).YData = [0 0 1 1 0 0]
      | sbobj.Groups(1).Signals(3).Name = 'recycling'
      | sbobj.Groups(1).Signals(3).XData = [0 6000 6000 8300 8300 8700 9150 14000]
      | sbobj.Groups(1).Signals(3).YData = [0 0 1 1 0 0 0 0]
      | sbobj.Groups(1).TimeRange = [0 14000]
      | sbobj.Groups(2).Name = 'Fan Temperature'
      | sbobj.Groups(2).Signals(1).Name = 'T_ext'
      | sbobj.Groups(2).Signals(1).XData = [0 100000]
      | sbobj.Groups(2).Signals(1).YData = [35 35]
      | sbobj.Groups(2).Signals(2).Name = 'door'
      | sbobj.Groups(2).Signals(2).XData = [0 100000]
      | sbobj.Groups(2).Signals(2).YData = [0 0]
      | sbobj.Groups(2).Signals(3).Name = 'recycling'
      | sbobj.Groups(2).Signals(3).XData = [0 100000]
      | sbobj.Groups(2).Signals(3).YData = [0 0]
      | sbobj.Groups(2).TimeRange = [0 100000]
      | sbobj.Groups(3).Name = 'Disturbances'
      | sbobj.Groups(3).Signals(1).Name = 'T_ext'
      | sbobj.Groups(3).Signals(1).XData = [0 100000]
      | sbobj.Groups(3).Signals(1).YData = [35 35]
      | sbobj.Groups(3).Signals(2).Name = 'door'
      | sbobj.Groups(3).Signals(2).XData = [0 20000 30000 40000 100000]
      | sbobj.Groups(3).Signals(2).YData = [0 0 1 0 0]
      | sbobj.Groups(3).Signals(3).Name = 'recycling'
      | sbobj.Groups(3).Signals(3).XData = [0 60000 60000 80000 80000 100000]
      | sbobj.Groups(3).Signals(3).YData = [0 0 0.5 0.5 0 0]
      | sbobj.Groups(3).TimeRange = [0 100000]
  T_ext : Outport  Tag=STV Outport  VectorParamsAs1DForOutWhenUnconnected=off
  door : Outport  Tag=STV Outport  Port=2  VectorParamsAs1DForOutWhenUnconnected=off
  recycling : Outport  Tag=STV Outport  Port=3  VectorParamsAs1DForOutWhenUnconnected=off
  wires:
  FromWs/1 -> Demux/1
  Demux/1 -> T_ext/1
  Demux/2 -> door/1
  Demux/3 -> recycling/1
